simulink model "sampleModel2065"  (R2023a)
settings: Solver=VariableStepAuto  StartTime=0.0  StopTime=10.0  RelTol=1e-3
libraries: hdlsllib x5, simulink x2
settings Model: Creator=user1  LastModifiedBy=user1

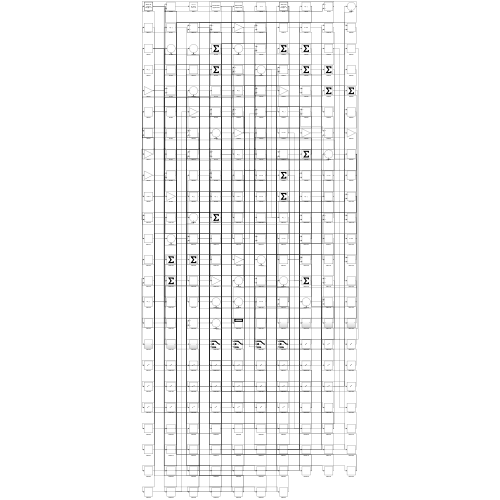
[thumbnail: Simulink's stored preview of the top-level diagram]
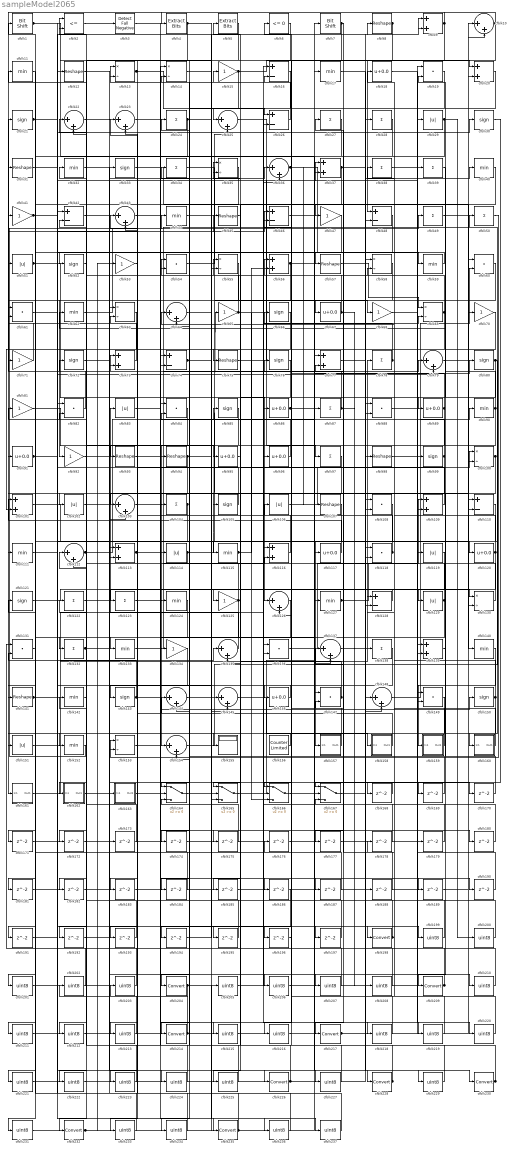
== system sampleModel2065 ==
  cfblk1 : hdlsllib/Logic and Bit Operations/Bit Shift  mode=Shift Left Logical  N=0
  cfblk{10,22..23,25,36,43,64,79,103,112,126,135,137,144..145,148,154} (17 alike) : Sum  Inputs=|++
  cfblk{13..14,35,55,58,63,69,100,130,153} (10 alike) : Product  Inputs=*/  RndMeth=Zero  SaturateOnIntegerOverflow=on
  cfblk{9,20,37,56,73,77,101,109,113,116,139} (11 alike) : Sum
  cfblk{29,51,83,102,106,114,119,129,151} (9 alike) : Abs  SaturateOnIntegerOverflow=off
  cfblk{24,27..28,34,38..39,49..50,78,87,97,104,122..123,132,138} (16 alike) : Sum  Inputs=+
  cfblk{21,30,33,52,66,72,76,80,85,99,105,121,143,150} (14 alike) : Signum
  cfblk{8,12,31,45,57,75,93..94,98,107,141} (11 alike) : Reshape
  cfblk{19,54,60..61,82,84,88,108,118,131,136,147,149} (13 alike) : DotProduct  OutDataTypeStr=Inherit: Inherit via internal rule
  cfblk{11,17,32,40,44,59,62,90,111,115,124,127,133,140,142,152} (16 alike) : MinMax
  cfblk{16,26,42,46,48,74,110,128} (8 alike) : Sum  Inputs=+-
  cfblk{18,67,86,89,91,95..96,117,120,146} (10 alike) : Bias  Bias=0.0  SaturateOnIntegerOverflow=off
  cfblk{15,41,47,53,65,68,70..71,81,92,125,134} (12 alike) : Gain
  cfblk155 : Display
  cfblk156 : hdlsllib/Sources/Counter Limited  uplimit=7  tsamp=-1
  cfblk157 : Subsystem
      settings: LibrarySourceBlock=|
      | hdlsllib/Ports &
      | Subsystems/Subsystem
  cfblk158 : Subsystem
      settings: LibrarySourceBlock=|
      | hdlsllib/Ports &
      | Subsystems/Subsystem
  cfblk159 : Subsystem
      settings: LibrarySourceBlock=|
      | hdlsllib/Ports &
      | Subsystems/Subsystem
  cfblk160 : Subsystem
      settings: LibrarySourceBlock=|
      | hdlsllib/Ports &
      | Subsystems/Subsystem
  cfblk161 : Subsystem
      settings: LibrarySourceBlock=|
      | hdlsllib/Ports &
      | Subsystems/Subsystem
  cfblk162 : Subsystem
      settings: LibrarySourceBlock=|
      | hdlsllib/Ports &
      | Subsystems/Subsystem
  cfblk163 : Subsystem
      settings: LibrarySourceBlock=|
      | hdlsllib/Ports &
      | Subsystems/Subsystem
  cfblk{164..167} (4 alike) : Switch  SaturateOnIntegerOverflow=off  InputSameDT=off
  cfblk{168..197} (30 alike) : Delay  SampleTime=1
  cfblk{198,204,209,214,217,226,228,230,232,235} (10 alike) : DataTypeConversion  SaturateOnIntegerOverflow=off  RndMeth=Floor
  cfblk{199..203,205..208,210..213,215..216,218..225,227,229,231,233..234,236..237} (30 alike) : DataTypeConversion  OutDataTypeStr=uint8  SaturateOnIntegerOverflow=off  RndMeth=Floor
  cfblk2 : RelationalOperator  Operator=<=  OutDataTypeStr=boolean  InputSameDT=off
  cfblk3 : hdlsllib/Logic and Bit Operations/Detect Fall Negative  vinit=0  OutDataTypeStr=boolean
  cfblk4 : simulink/Logic and Bit Operations/Extract Bits  bitsToExtract=Upper half  numBits=8  bitIdxRange=[0 7]  outScalingMode=Preserve fixed-point scaling
      settings: LibrarySourceBlock=|
      | hdlsllib/Logic and Bit
      | Operations/Extract Bits
  cfblk5 : simulink/Logic and Bit Operations/Extract Bits  bitsToExtract=Upper half  numBits=8  bitIdxRange=[0 7]  outScalingMode=Preserve fixed-point scaling
      settings: LibrarySourceBlock=|
      | hdlsllib/Logic and Bit
      | Operations/Extract Bits
  cfblk6 : hdlsllib/Logic and Bit Operations/Compare To Zero  relop=<=  OutDataTypeStr=boolean
  cfblk7 : hdlsllib/Logic and Bit Operations/Bit Shift  mode=Shift Left Logical  N=0
  wires:
  cfblk34/1 -> cfblk68/1
  cfblk26/1 -> cfblk13/1
  cfblk135/1 -> cfblk83/1
  cfblk56/1 -> cfblk166/2, cfblk189/1, cfblk190/1
  cfblk25/1 -> cfblk97/1
  cfblk151/1 -> cfblk78/1
  cfblk85/1 -> cfblk154/1
  cfblk51/1 -> cfblk126/1, cfblk9/1
  cfblk57/1 -> cfblk69/1
  cfblk106/1 -> cfblk100/1
  cfblk154/1 -> cfblk50/1
  cfblk60/1 -> cfblk92/1
  cfblk110/1 -> cfblk157/1(In1)
  cfblk44/1 -> cfblk117/1
  cfblk118/1 -> cfblk27/1, cfblk41/1
  cfblk121/1 -> cfblk130/1
  cfblk152/1 -> cfblk44/1
  cfblk148/1 -> cfblk90/1
  cfblk136/1 -> cfblk109/1
  cfblk50/1 -> cfblk153/1
  cfblk114/1 -> cfblk65/1, cfblk113/2
  cfblk112/1 -> cfblk7/1, cfblk129/1
  cfblk143/1 -> cfblk121/1, cfblk210/1
  cfblk49/1 -> cfblk140/1
  cfblk9/1 -> cfblk161/1(In1), cfblk52/1
  cfblk87/1 -> cfblk2/2, cfblk208/1
  cfblk144/1 -> cfblk198/1
  cfblk29/1 -> cfblk116/1, cfblk200/1
  cfblk91/1 -> cfblk30/1, cfblk45/1
  cfblk65/1 -> cfblk2/1, cfblk166/3, cfblk218/1
  cfblk128/1 -> cfblk125/1
  cfblk161/1(Out1) -> cfblk135/1
  cfblk133/1 -> cfblk116/2
  cfblk149/1 -> cfblk151/1
  cfblk98/1 -> cfblk60/2
  cfblk79/1 -> cfblk110/1
  cfblk15/1 -> cfblk20/1, cfblk194/1
  cfblk102/1 -> cfblk33/1
  cfblk101/1 -> cfblk130/2
  cfblk166/1 -> cfblk87/1
  cfblk32/1 -> cfblk226/1
  cfblk40/1 -> cfblk75/1
  cfblk82/1 -> cfblk21/1
  cfblk76/1 -> cfblk165/1
  cfblk13/1 -> cfblk25/1, cfblk137/2
  cfblk28/1 -> cfblk204/1
  cfblk71/1 -> cfblk31/1
  cfblk45/1 -> cfblk105/1
  cfblk96/1 -> cfblk15/1
  cfblk80/1 -> cfblk160/1(In1), cfblk96/1, cfblk120/1, cfblk225/1
  cfblk21/1 -> cfblk59/1, cfblk145/2, cfblk195/1, cfblk227/1
  cfblk10/1 -> cfblk48/1, cfblk4/1
  cfblk62/1 -> cfblk49/1
  cfblk77/1 -> cfblk40/1
  cfblk156/1 -> cfblk152/1
  cfblk1/1 -> cfblk147/1, cfblk145/1, cfblk79/2
  cfblk31/1 -> cfblk12/1
  cfblk99/1 -> cfblk54/1, cfblk177/1
  cfblk8/1 -> cfblk192/1, cfblk193/1
  cfblk125/1 -> cfblk81/1, cfblk183/1, cfblk185/1
  cfblk94/1 -> cfblk102/1, cfblk8/1
  cfblk4/1 -> cfblk103/1, cfblk86/1, cfblk186/1
  cfblk68/1 -> cfblk29/1
  cfblk95/1 -> cfblk5/1
  cfblk24/1 -> cfblk112/2, cfblk61/1, cfblk47/1
  cfblk74/1 -> cfblk197/1, cfblk236/1
  cfblk73/1 -> cfblk51/1
  cfblk164/1 -> cfblk36/1
  cfblk48/1 -> cfblk135/2
  cfblk59/1 -> cfblk57/1
  cfblk103/1 -> cfblk79/1
  cfblk75/1 -> cfblk19/1
  cfblk14/1 -> cfblk26/1
  cfblk120/1 -> cfblk18/1, cfblk216/1
  cfblk123/1 -> cfblk20/2
  cfblk69/1 -> cfblk46/2, cfblk196/1
  cfblk165/1 -> cfblk80/1
  cfblk18/1 -> cfblk119/1
  cfblk64/1 -> cfblk127/1
  cfblk63/1 -> cfblk232/1
  cfblk150/1 -> cfblk167/1, cfblk128/1
  cfblk70/1 -> cfblk162/1(In1)
  cfblk111/1 -> cfblk100/2
  cfblk53/1 -> cfblk93/1
  cfblk147/1 -> cfblk85/1, cfblk146/1
  cfblk39/1 -> cfblk89/1
  cfblk104/1 -> cfblk141/1, cfblk231/1
  cfblk37/1 -> cfblk48/2, cfblk115/1
  cfblk140/1 -> cfblk159/1(In1)
  cfblk17/1 -> cfblk230/1
  cfblk36/1 -> cfblk118/2, cfblk107/1
  cfblk159/1(Out1) -> cfblk64/1
  cfblk160/1(Out1) -> cfblk38/1
  cfblk105/1 -> cfblk73/1
  cfblk167/1 -> cfblk98/1
  cfblk20/1 -> cfblk94/1
  cfblk7/1 -> cfblk67/1, cfblk132/1, cfblk166/1
  cfblk97/1 -> cfblk111/1
  cfblk153/1 -> cfblk150/1
  cfblk141/1 -> cfblk69/2, cfblk46/1
  cfblk54/1 -> cfblk25/2
  cfblk41/1 -> cfblk114/1, cfblk37/1
  cfblk116/1 -> cfblk72/1
  cfblk89/1 -> cfblk16/2, cfblk172/1
  cfblk92/1 -> cfblk104/1
  cfblk130/1 -> cfblk11/1
  cfblk137/1 -> cfblk148/2
  cfblk27/1 -> cfblk74/2
  cfblk90/1 -> cfblk124/1, cfblk62/1
  cfblk119/1 -> cfblk123/1
  cfblk33/1 -> cfblk70/1
  cfblk122/1 -> cfblk228/1
  cfblk145/1 -> cfblk158/1(In1)
  cfblk127/1 -> cfblk39/1, cfblk9/2
  cfblk129/1 -> cfblk34/1, cfblk165/3
  cfblk146/1 -> cfblk143/1
  cfblk108/1 -> cfblk214/1
  cfblk58/1 -> cfblk217/1
  cfblk100/1 -> cfblk133/1, cfblk169/1, cfblk171/1
  cfblk157/1(Out1) -> cfblk66/1
  cfblk2/1 -> cfblk3/1
  cfblk55/1 -> cfblk91/1
  cfblk126/1 -> cfblk134/1
  cfblk12/1 -> cfblk110/2
  cfblk19/1 -> cfblk136/2
  cfblk115/1 -> cfblk155/1, cfblk56/2
  cfblk86/1 -> cfblk6/1, cfblk128/2
  cfblk117/1 -> cfblk101/1
  cfblk23/1 -> cfblk235/1
  cfblk66/1 -> cfblk101/2
  cfblk139/1 -> cfblk209/1
  cfblk16/1 -> cfblk164/1
  cfblk67/1 -> cfblk22/1, cfblk138/1
  cfblk132/1 -> cfblk163/1(In1), cfblk222/1
  cfblk52/1 -> cfblk22/2
  cfblk81/1 -> cfblk95/1
  cfblk158/1(Out1) -> cfblk43/1
  cfblk78/1 -> cfblk71/1, cfblk56/1
  cfblk109/1 -> cfblk55/1
  cfblk162/1(Out1) -> cfblk35/1
  cfblk113/1 -> cfblk215/1, cfblk219/1
  cfblk30/1 -> cfblk168/1
  cfblk168/1 -> cfblk167/2
  cfblk169/1 -> cfblk13/2
  cfblk72/1 -> cfblk170/1
  cfblk170/1 -> cfblk19/2
  cfblk171/1 -> cfblk55/2
  cfblk172/1 -> cfblk109/2
  cfblk22/1 -> cfblk173/1
  cfblk173/1 -> cfblk112/1
  cfblk138/1 -> cfblk174/1
  cfblk174/1 -> cfblk136/1
  cfblk163/1(Out1) -> cfblk175/1
  cfblk175/1 -> cfblk154/2
  cfblk176/1 -> cfblk118/1
  cfblk177/1 -> cfblk137/1
  cfblk178/1 -> cfblk77/2
  cfblk38/1 -> cfblk179/1
  cfblk179/1 -> cfblk16/1
  cfblk83/1 -> cfblk180/1
  cfblk180/1 -> cfblk147/2
  cfblk11/1 -> cfblk181/1
  cfblk181/1 -> cfblk148/1
  cfblk6/1 -> cfblk182/1
  cfblk182/1 -> cfblk14/1
  cfblk183/1 -> cfblk10/1
  cfblk5/1 -> cfblk184/1
  cfblk184/1 -> cfblk1/1
  cfblk185/1 -> cfblk26/2
  cfblk43/1 -> cfblk187/1
  cfblk187/1 -> cfblk74/1
  cfblk188/1 -> cfblk167/3
  cfblk189/1 -> cfblk60/1
  cfblk190/1 -> cfblk149/1
  cfblk35/1 -> cfblk191/1
  cfblk192/1 -> cfblk153/2
  cfblk193/1 -> cfblk82/2
  cfblk194/1 -> cfblk165/2
  cfblk195/1 -> cfblk73/2
  cfblk196/1 -> cfblk126/2
  cfblk197/1 -> cfblk164/2
  cfblk198/1 -> cfblk178/1, cfblk106/1
  cfblk3/1 -> cfblk199/1
  cfblk199/1 -> cfblk144/1
  cfblk200/1 -> cfblk144/2
  cfblk131/1 -> cfblk201/1
  cfblk201/1 -> cfblk113/1
  cfblk202/1 -> cfblk131/1
  cfblk203/1 -> cfblk131/2
  cfblk204/1 -> cfblk203/1, cfblk36/2, cfblk14/2
  cfblk205/1 -> cfblk28/1
  cfblk42/1 -> cfblk206/1
  cfblk206/1 -> cfblk99/1
  cfblk93/1 -> cfblk207/1
  cfblk207/1 -> cfblk42/1
  cfblk208/1 -> cfblk42/2
  cfblk209/1 -> cfblk54/2, cfblk64/2
  cfblk210/1 -> cfblk139/1
  cfblk124/1 -> cfblk211/1
  cfblk211/1 -> cfblk139/2
  cfblk142/1 -> cfblk212/1
  cfblk212/1 -> cfblk103/2
  cfblk107/1 -> cfblk213/1
  cfblk213/1 -> cfblk142/1
  cfblk214/1 -> cfblk43/2, cfblk10/2
  cfblk215/1 -> cfblk108/1
  cfblk216/1 -> cfblk108/2
  cfblk217/1 -> cfblk188/1, cfblk149/2
  cfblk218/1 -> cfblk58/1
  cfblk219/1 -> cfblk58/2
  cfblk88/1 -> cfblk220/1
  cfblk220/1 -> cfblk176/1
  cfblk47/1 -> cfblk221/1
  cfblk221/1 -> cfblk88/1
  cfblk222/1 -> cfblk88/2
  cfblk84/1 -> cfblk223/1
  cfblk223/1 -> cfblk202/1
  cfblk61/1 -> cfblk224/1
  cfblk224/1 -> cfblk84/1
  cfblk225/1 -> cfblk84/2
  cfblk226/1 -> cfblk37/2, cfblk24/1
  cfblk227/1 -> cfblk32/1
  cfblk228/1 -> cfblk35/2, cfblk76/1
  cfblk46/1 -> cfblk229/1
  cfblk229/1 -> cfblk122/1
  cfblk230/1 -> cfblk164/3, cfblk77/1
  cfblk231/1 -> cfblk17/1
  cfblk232/1 -> cfblk205/1, cfblk53/1
  cfblk134/1 -> cfblk233/1
  cfblk233/1 -> cfblk63/1
  cfblk186/1 -> cfblk234/1
  cfblk234/1 -> cfblk63/2
  cfblk235/1 -> cfblk61/2, cfblk82/1
  cfblk236/1 -> cfblk23/1
  cfblk191/1 -> cfblk237/1
  cfblk237/1 -> cfblk23/2

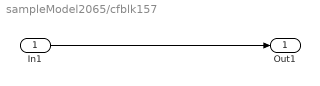
== system sampleModel2065/cfblk157 ==
  In1 : Inport
  Out1 : Outport
  wires:
  In1/1 -> Out1/1

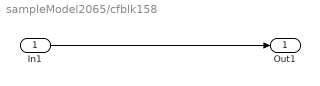
== system sampleModel2065/cfblk158 ==
  In1 : Inport
  Out1 : Outport
  wires:
  In1/1 -> Out1/1

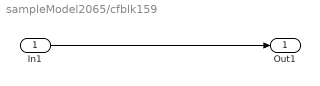
== system sampleModel2065/cfblk159 ==
  In1 : Inport
  Out1 : Outport
  wires:
  In1/1 -> Out1/1

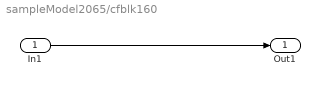
== system sampleModel2065/cfblk160 ==
  In1 : Inport
  Out1 : Outport
  wires:
  In1/1 -> Out1/1

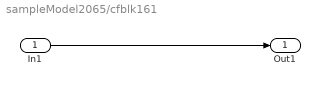
== system sampleModel2065/cfblk161 ==
  In1 : Inport
  Out1 : Outport
  wires:
  In1/1 -> Out1/1

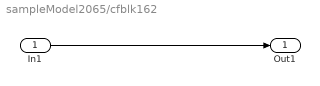
== system sampleModel2065/cfblk162 ==
  In1 : Inport
  Out1 : Outport
  wires:
  In1/1 -> Out1/1

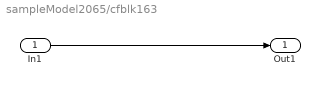
== system sampleModel2065/cfblk163 ==
  In1 : Inport
  Out1 : Outport
  wires:
  In1/1 -> Out1/1
